simulink model "ss_modelo"  (R2021a)
settings: Solver=VariableStepAuto  StartTime=0.0  StopTime=120  RelTol=1e-3
values from neighbouring files (symbols this model uses):
  sys = n4sid(data)    [linealizacion.m]    (also in linealizacion_0.m)
settings Model: Creator=Seb  LastModifiedBy=Seb

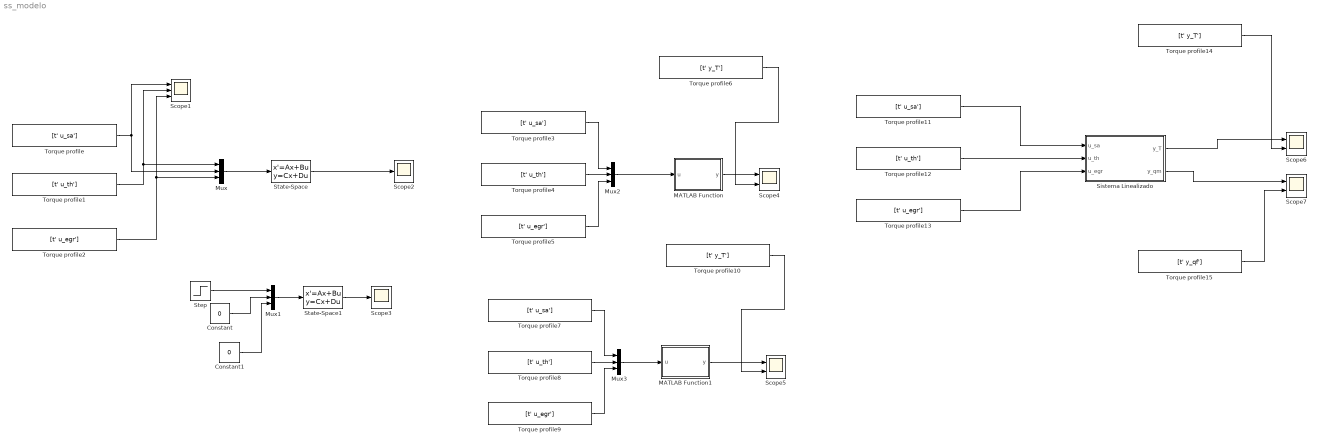
== system ss_modelo ==
  Constant : Constant  Value=0
  Constant1 : Constant  Value=0
  MATLAB Function : MATLAB Function  TreatAsAtomicUnit=on
  MATLAB Function1 : MATLAB Function  TreatAsAtomicUnit=on
  Mux{,1..3} (4 alike) : Mux  Inputs=3
  Scope1 : Scope  NumInputPorts=3
  Scope2 : Scope
  Scope3 : Scope
  Scope{4..7} (4 alike) : Scope  NumInputPorts=2
  Sistema Linealizado : Subsystem
  State-Space : StateSpace  A=sys.A  B=sys.B  C=sys.C  D=sys.D  InitialCondition=0
  State-Space1 : StateSpace  A=sys.A  B=sys.B  C=sys.C  D=sys.D  InitialCondition=0
  Step : Step  SampleTime=0
  Torque profile{,3,7,11} (4 alike) : FromWorkspace  VariableName=[t' u_sa']  SampleTime=-1  OutputAfterFinalValue=Holding final value
  Torque profile{1,4,8,12} (4 alike) : FromWorkspace  VariableName=[t' u_th']  SampleTime=-1  OutputAfterFinalValue=Holding final value
  Torque profile10 : FromWorkspace  VariableName=[t' y_T']  SampleTime=-1  OutputAfterFinalValue=Holding final value
  Torque profile{2,5,9,13} (4 alike) : FromWorkspace  VariableName=[t' u_egr']  SampleTime=-1  OutputAfterFinalValue=Holding final value
  Torque profile14 : FromWorkspace  VariableName=[t' y_T']  SampleTime=-1  OutputAfterFinalValue=Holding final value
  Torque profile15 : FromWorkspace  VariableName=[t' y_qf']  SampleTime=-1  OutputAfterFinalValue=Holding final value
  Torque profile6 : FromWorkspace  VariableName=[t' y_T']  SampleTime=-1  OutputAfterFinalValue=Holding final value
  wires:
  Mux/1 -> State-Space/1
  Torque profile/1 -> Mux/2, Scope1/1
  Torque profile1/1 -> Mux/1, Scope1/2
  Torque profile2/1 -> Mux/3, Scope1/3
  State-Space/1 -> Scope2/1
  State-Space1/1 -> Scope3/1
  Mux1/1 -> State-Space1/1
  Step/1 -> Mux1/1
  Constant/1 -> Mux1/2
  Constant1/1 -> Mux1/3
  MATLAB Function/1(y) -> Scope4/1
  Mux2/1 -> MATLAB Function/1(u)
  Torque profile3/1 -> Mux2/1
  Torque profile4/1 -> Mux2/2
  Torque profile5/1 -> Mux2/3
  Torque profile6/1 -> Scope4/2
  Torque profile10/1 -> Scope5/2
  Torque profile9/1 -> Mux3/3
  Torque profile8/1 -> Mux3/2
  Torque profile7/1 -> Mux3/1
  Mux3/1 -> MATLAB Function1/1(u)
  MATLAB Function1/1(y) -> Scope5/1
  Torque profile14/1 -> Scope6/2
  Torque profile15/1 -> Scope7/2
  Torque profile11/1 -> Sistema Linealizado/1(u_sa)
  Torque profile12/1 -> Sistema Linealizado/2(u_th)
  Torque profile13/1 -> Sistema Linealizado/3(u_egr)
  Sistema Linealizado/1(y_T) -> Scope6/1
  Sistema Linealizado/2(y_qm) -> Scope7/1

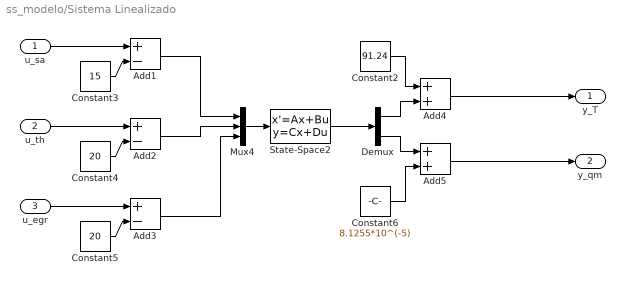
== system ss_modelo/Sistema Linealizado ==
  u_sa : Inport
  u_th : Inport  Port=2
  u_egr : Inport  Port=3
  Add1 : Sum  Inputs=+-
  Add2 : Sum  Inputs=+-
  Add3 : Sum  Inputs=+-
  Add4 : Sum
  Add5 : Sum
  Constant2 : Constant  Value=91.24
  Constant3 : Constant  Value=15
  Constant4 : Constant  Value=20
  Constant5 : Constant  Value=20
  Constant6 : Constant  Value=8.1255*10^(-5)
  Demux : Demux  Outputs=2
  Mux4 : Mux  Inputs=3
  State-Space2 : StateSpace  A=[0]  B=[0 0 0]  C=[0;0]  D=[0.1577 6.775 0.2081; 5.8115*10^(-12) 4.289*10^(-6) 1.4775*10^(-8)]  InitialCondition=0
  y_T : Outport
  y_qm : Outport  Port=2
  wires:
  u_sa/1 -> Add1/1
  Constant3/1 -> Add1/2
  Constant2/1 -> Add4/1
  State-Space2/1 -> Demux/1
  Demux/1 -> Add4/2
  Add3/1 -> Mux4/3
  Constant5/1 -> Add3/2
  Mux4/1 -> State-Space2/1
  Add1/1 -> Mux4/1
  Add2/1 -> Mux4/2
  Constant6/1 -> Add5/2
  Constant4/1 -> Add2/2
  Demux/2 -> Add5/1
  Add5/1 -> y_qm/1
  u_egr/1 -> Add3/1
  u_th/1 -> Add2/1
  Add4/1 -> y_T/1

== matlab function ss_modelo/MATLAB Function ==
  data: u input; y output
function y = fcn(u)
u_sa = u(1);
u_th = u(2);
u_egr = u(3);
y0 = 97.3;
u_sa0 = 20;
y_sa = 0.1043;
u_th0 = 17.5;
y_th = 10.39;
u_egr0 = 12.5;
y_egr = 0.25585;
y = y0 + y_sa*(u_sa-u_sa0) + y_th*(u_th-u_th0) + y_egr*(u_egr-u_egr0);

== matlab function ss_modelo/MATLAB Function1 ==
  data: u input; y output
function y = fcn(u)
u_sa = u(1);
u_th = u(2);
u_egr = u(3);
y0 = 91.24;
u_sa0 = 15;
y_sa = 0.1577;
u_th0 = 20;
y_th = 6.775;
u_egr0 = 20;
y_egr = 0.2081;
y = y0 + y_sa*(u_sa-u_sa0) + y_th*(u_th-u_th0) + y_egr*(u_egr-u_egr0);
